simulink model "E5_2_Harmonicas"  (R2018a)
settings: Solver=VariableStepAuto  StartTime=0.0  StopTime=1  RelTol=1e-3
libraries: powerlib x29
settings Model: Creator=Rafael Pavan  LastModifiedBy=Rafael Pavan

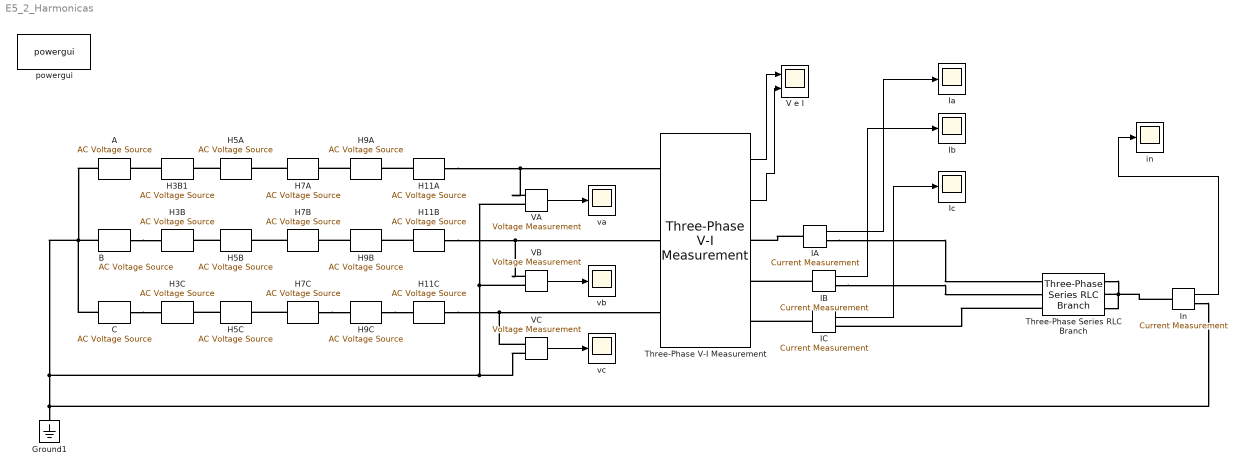
== system E5_2_Harmonicas ==
  A : powerlib/Electrical Sources/AC Voltage Source  Amplitude=179.605  Phase=0  Frequency=60  SampleTime=0  Measurements=None  BusType=PV  Pref=100e4  Qref=0  Qmin=-inf  Qmax=+inf
  B : powerlib/Electrical Sources/AC Voltage Source  Amplitude=179.605  Phase=-120  Frequency=60  SampleTime=0  Measurements=None  BusType=PV  Pref=100e4  Qref=0  Qmin=-inf  Qmax=+inf
  C : powerlib/Electrical Sources/AC Voltage Source  Amplitude=179.605  Phase=120  Frequency=60  SampleTime=0  Measurements=None  BusType=PV  Pref=100e4  Qref=0  Qmin=-inf  Qmax=+inf
  Ground1 : powerlib/Elements/Ground  LConnTagsString=a
  H11A : powerlib/Electrical Sources/AC Voltage Source  Amplitude=179.605*2/100  Phase=0  Frequency=660  SampleTime=0  Measurements=None  BusType=PV  Pref=100e4  Qref=0  Qmin=-inf  Qmax=+inf
  H11B : powerlib/Electrical Sources/AC Voltage Source  Amplitude=179.605*2/100  Phase=-120*11  Frequency=660  SampleTime=0  Measurements=None  BusType=PV  Pref=100e4  Qref=0  Qmin=-inf  Qmax=+inf
  H11C : powerlib/Electrical Sources/AC Voltage Source  Amplitude=179.605*2/100  Phase=120*11  Frequency=660  SampleTime=0  Measurements=None  BusType=PV  Pref=100e4  Qref=0  Qmin=-inf  Qmax=+inf
  H3B : powerlib/Electrical Sources/AC Voltage Source  Amplitude=179.605*10/100  Phase=-120*3  Frequency=180  SampleTime=0  Measurements=None  BusType=PV  Pref=100e4  Qref=0  Qmin=-inf  Qmax=+inf
  H3B1 : powerlib/Electrical Sources/AC Voltage Source  Amplitude=179.605*10/100  Phase=0*3  Frequency=60*3  SampleTime=0  Measurements=None  BusType=PV  Pref=100e4  Qref=0  Qmin=-inf  Qmax=+inf
  H3C : powerlib/Electrical Sources/AC Voltage Source  Amplitude=179.605*10/100  Phase=120*3  Frequency=180  SampleTime=0  Measurements=None  BusType=PV  Pref=100e4  Qref=0  Qmin=-inf  Qmax=+inf
  H5A : powerlib/Electrical Sources/AC Voltage Source  Amplitude=179.605*5/100  Phase=0  Frequency=300  SampleTime=0  Measurements=None  BusType=PV  Pref=100e4  Qref=0  Qmin=-inf  Qmax=+inf
  H5B : powerlib/Electrical Sources/AC Voltage Source  Amplitude=179.605*5/100  Phase=-120*5  Frequency=300  SampleTime=0  Measurements=None  BusType=PV  Pref=100e4  Qref=0  Qmin=-inf  Qmax=+inf
  H5C : powerlib/Electrical Sources/AC Voltage Source  Amplitude=179.605*5/100  Phase=120*5  Frequency=300  SampleTime=0  Measurements=None  BusType=PV  Pref=100e4  Qref=0  Qmin=-inf  Qmax=+inf
  H7A : powerlib/Electrical Sources/AC Voltage Source  Amplitude=179.605*3/100  Phase=0  Frequency=420  SampleTime=0  Measurements=None  BusType=PV  Pref=100e4  Qref=0  Qmin=-inf  Qmax=+inf
  H7B : powerlib/Electrical Sources/AC Voltage Source  Amplitude=179.605*3/100  Phase=-120*7  Frequency=420  SampleTime=0  Measurements=None  BusType=PV  Pref=100e4  Qref=0  Qmin=-inf  Qmax=+inf
  H7C : powerlib/Electrical Sources/AC Voltage Source  Amplitude=179.605*3/100  Phase=120*7  Frequency=420  SampleTime=0  Measurements=None  BusType=PV  Pref=100e4  Qref=0  Qmin=-inf  Qmax=+inf
  "H9A " : powerlib/Electrical Sources/AC Voltage Source  Amplitude=179.605*2/100  Phase=0  Frequency=540  SampleTime=0  Measurements=None  BusType=PV  Pref=100e4  Qref=0  Qmin=-inf  Qmax=+inf
  H9B : powerlib/Electrical Sources/AC Voltage Source  Amplitude=179.605*2/100  Phase=-120*9  Frequency=540  SampleTime=0  Measurements=None  BusType=PV  Pref=100e4  Qref=0  Qmin=-inf  Qmax=+inf
  H9C : powerlib/Electrical Sources/AC Voltage Source  Amplitude=179.605*2/100  Phase=120*9  Frequency=540  SampleTime=0  Measurements=None  BusType=PV  Pref=100e4  Qref=0  Qmin=-inf  Qmax=+inf
  IA : powerlib/Measurements/Current Measurement  PhasorSimulation=off  OutputType=Complex  PSBequivalent=0
  IB : powerlib/Measurements/Current Measurement  PhasorSimulation=off  OutputType=Complex  PSBequivalent=0
  IC : powerlib/Measurements/Current Measurement  PhasorSimulation=off  OutputType=Complex  PSBequivalent=0
  Ia : Scope
  Ib : Scope
  "Ic " : Scope
  In : powerlib/Measurements/Current Measurement  PhasorSimulation=off  OutputType=Complex  PSBequivalent=0
  Three-Phase Series RLC Branch : powerlib/Elements/Three-Phase Series RLC Branch  LConnTagsString=A|B|C  RConnTagsString=A|B|C  BranchType=RLC  Resistance=1  Inductance=1e-4  Capacitance=1e-4  Measurements=None
  Three-Phase V-I Measurement : powerlib/Measurements/Three-Phase V-I Measurement  VoltageMeasurement=phase-to-ground  SetLabelV=off  LabelV=Vabc  Vpu=off  VpuLL=off  CurrentMeasurement=yes  SetLabelI=off  LabelI=Iabc  Ipu=off  Pbase=100e6  Vbase=500e3  OutputType=Complex  PhasorSimulation=off  PSBequivalent=0
  V e I : Scope  NumInputPorts=2
  VA : powerlib/Measurements/Voltage Measurement  PhasorSimulation=off  OutputType=Complex  PSBequivalent=0
  VB : powerlib/Measurements/Voltage Measurement  PhasorSimulation=off  OutputType=Complex  PSBequivalent=0
  VC : powerlib/Measurements/Voltage Measurement  PhasorSimulation=off  OutputType=Complex  PSBequivalent=0
  in : Scope
  powergui : powerlib/powergui  Priority=1  SimulationMode=Continuous  SampleTime=50e-6  frequency=60  Iterations=50  frequencyindice=60  Pbase=100e6  ErrMax=1e-4  UnitsV=kV  UnitsW=MW  buscounter=0  FunctionMessages=on  echomessages=off  EnableUseOfTLC=off  CurrentSourceSwitches=off  DisableSnubberDevices=off  DisableRonSwitches=off  DisableVfSwitches=off  DisplayEquations=off  SolverType=Tustin/Backward Euler (TBE)  Interpol=off  ExternalGateDelay=off  methode=off  Ts=100  x0status=blocks  SPID=on  SwTol=0  HookPort=off  RestoreLinks=warning  ResistiveCurrentMeasurement=off  Frange=[0:2:500]  Ylog=off  Xlog=on  ShowGrid=off  save=off  variable=ZData  structure=ia  ZoomFFT=off  StartTime=0.2  cycles=12  DisplayStyle=1  fundamental=60  FreqAxis=off  MaxFrequency=1000  frequencyindicesteady=1  RmsSteady=2  display=off
  va : Scope
  vb : Scope
  vc : Scope
  wires:
  VA/1 -> va/1
  VB/1 -> vb/1
  VC/1 -> vc/1
  Three-Phase V-I Measurement/1 -> V e I/1
  IA/1 -> Ia/1
  IB/1 -> Ib/1
  IC/1 -> "Ic "/1
  Three-Phase V-I Measurement/2 -> V e I/2
  In/1 -> in/1
  connections:
  A/LConn1 -- C/LConn1 -- B/LConn1 -- VA/LConn2 -- VB/LConn2 -- VC/LConn2 -- In/RConn1 -- Ground1/LConn1
  H3B1/LConn1 -- A/RConn1
  B/RConn1 -- H3B/LConn1
  C/RConn1 -- H3C/LConn1
  H11C/RConn1 -- VC/LConn1 -- Three-Phase V-I Measurement/LConn3
  H11B/RConn1 -- VB/LConn1 -- Three-Phase V-I Measurement/LConn2
  H5A/LConn1 -- H3B1/RConn1
  H7B/LConn1 -- H5B/RConn1
  H5C/LConn1 -- H3C/RConn1
  H7A/LConn1 -- H5A/RConn1
  "H9A "/LConn1 -- H7A/RConn1
  H5B/LConn1 -- H3B/RConn1
  H11B/LConn1 -- H9B/RConn1
  H7C/LConn1 -- H5C/RConn1
  H9B/LConn1 -- H7B/RConn1
  H9C/RConn1 -- H11C/LConn1
  H11A/LConn1 -- "H9A "/RConn1
  H7C/RConn1 -- H9C/LConn1
  H11A/RConn1 -- VA/LConn1 -- Three-Phase V-I Measurement/LConn1
  IA/LConn1 -- Three-Phase V-I Measurement/RConn1
  IB/LConn1 -- Three-Phase V-I Measurement/RConn2
  IC/LConn1 -- Three-Phase V-I Measurement/RConn3
  Three-Phase Series RLC Branch/LConn3 -- IC/RConn1
  IB/RConn1 -- Three-Phase Series RLC Branch/LConn2
  IA/RConn1 -- Three-Phase Series RLC Branch/LConn1
  Three-Phase Series RLC Branch/RConn1 -- In/LConn1 -- Three-Phase Series RLC Branch/RConn3 -- Three-Phase Series RLC Branch/RConn2
